simulink model "rockTrackingModelOne"  (R2023b)
settings: Solver=VariableStepAuto  StartTime=0.0  StopTime=10.0  RelTol=1e-3
settings Model: Creator=leif  LastModifiedBy=leif

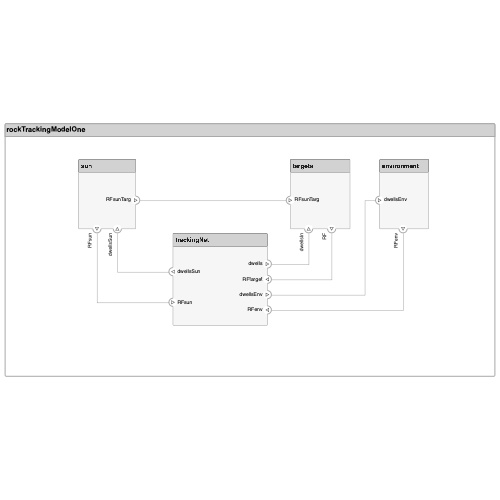
[thumbnail: Simulink's stored preview of the top-level diagram]
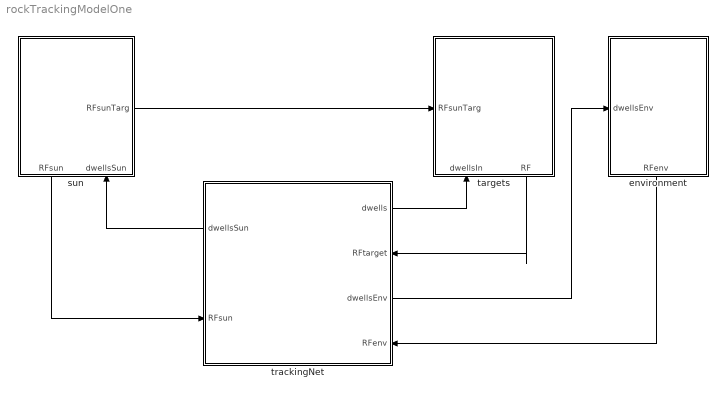
== system rockTrackingModelOne ==
  environment : Subsystem
      settings: PortSchema="{\"entries\":[{\"content\":{\"headerSize\":26,\"margin\":15,\"minimumSpacing\":25,\"sides\":[{\"content\":{\"connectorIds\":[\"In1\"]},\"type\":\"ConnectorPlacement.EquallySpacedRectSide\",\"uuid\":\"8862968b-5599-41d0-9291-c0c671b7ec34\"},{\"content\":{\"side\":\"RIGHT\"},\"type\":\"ConnectorPlacement.EquallySpacedRectSide\",\"uuid\":\"824bb606-5208-4b2e-9988-455833bc9c0f\"},{\"content\":{\"side\":\"TOP\"},\"type\":\"ConnectorPlacement.EquallySpacedRectSide\",\"uuid\":\"80947048-364c-4417-9b61-7a75165eca9d\"},{\"content\":{\"connectorIds\":[\"Out1\"],\"side\":\"BOTTOM\"},\"type\":\"ConnectorPlacement.EquallySpacedRectSide\",\"uuid\":\"629623b4-050a-43a5-9a7b-197cf824730b\"}]},\"type\":\"ConnectorPlacement.EquallySpacedConnector\",\"uuid\":\"bd0727a2-e7c6-4cf8-803d-4ba2eab1ab1b\"}],\"packageUris\":[\"http://schema.mathworks.com/mf0/Connector/R2020b\"],\"version\":\"1.0\"}"
  sun : Subsystem
      settings: PortSchema="{\"entries\":[{\"content\":{\"headerSize\":26,\"margin\":15,\"minimumSpacing\":25,\"sides\":[{\"content\":{},\"type\":\"ConnectorPlacement.EquallySpacedRectSide\",\"uuid\":\"8862968b-5599-41d0-9291-c0c671b7ec34\"},{\"content\":{\"connectorIds\":[\"Out2\"],\"side\":\"RIGHT\"},\"type\":\"ConnectorPlacement.EquallySpacedRectSide\",\"uuid\":\"824bb606-5208-4b2e-9988-455833bc9c0f\"},{\"content\":{\"side\":\"TOP\"},\"type\":\"ConnectorPlacement.EquallySpacedRectSide\",\"uuid\":\"80947048-364c-4417-9b61-7a75165eca9d\"},{\"content\":{\"connectorIds\":[\"Out1\",\"In1\"],\"side\":\"BOTTOM\"},\"type\":\"ConnectorPlacement.EquallySpacedRectSide\",\"uuid\":\"9527848b-f77a-4aa4-b4b8-8e4a885b14ab\"}]},\"type\":\"ConnectorPlacement.EquallySpacedConnector\",\"uuid\":\"bd0727a2-e7c6-4cf8-803d-4ba2eab1ab1b\"}],\"packageUris\":[\"http://schema.mathworks.com/mf0/Connector/R2020b\"],\"version\":\"1.0\"}"
  targets : Subsystem
      settings: PortSchema="{\"entries\":[{\"content\":{\"headerSize\":26,\"margin\":15,\"minimumSpacing\":25,\"sides\":[{\"content\":{\"connectorIds\":[\"In2\"]},\"type\":\"ConnectorPlacement.EquallySpacedRectSide\",\"uuid\":\"8862968b-5599-41d0-9291-c0c671b7ec34\"},{\"content\":{\"side\":\"RIGHT\"},\"type\":\"ConnectorPlacement.EquallySpacedRectSide\",\"uuid\":\"824bb606-5208-4b2e-9988-455833bc9c0f\"},{\"content\":{\"side\":\"TOP\"},\"type\":\"ConnectorPlacement.EquallySpacedRectSide\",\"uuid\":\"80947048-364c-4417-9b61-7a75165eca9d\"},{\"content\":{\"connectorIds\":[\"In1\",\"Out1\"],\"side\":\"BOTTOM\"},\"type\":\"ConnectorPlacement.EquallySpacedRectSide\",\"uuid\":\"629623b4-050a-43a5-9a7b-197cf824730b\"}]},\"type\":\"ConnectorPlacement.EquallySpacedConnector\",\"uuid\":\"bd0727a2-e7c6-4cf8-803d-4ba2eab1ab1b\"}],\"packageUris\":[\"http://schema.mathworks.com/mf0/Connector/R2020b\"],\"version\":\"1.0\"}"
  trackingNet : Subsystem
      settings: PortSchema="{\"entries\":[{\"content\":{\"headerSize\":26,\"margin\":15,\"minimumSpacing\":25,\"sides\":[{\"content\":{\"connectorIds\":[\"Out2\",\"In1\"]},\"type\":\"ConnectorPlacement.EquallySpacedRectSide\",\"uuid\":\"8862968b-5599-41d0-9291-c0c671b7ec34\"},{\"content\":{\"connectorIds\":[\"Out1\",\"In3\",\"Out3\",\"In2\"],\"side\":\"RIGHT\"},\"type\":\"ConnectorPlacement.EquallySpacedRectSide\",\"uuid\":\"824bb606-5208-4b2e-9988-455833bc9c0f\"},{\"content\":{\"side\":\"TOP\"},\"type\":\"ConnectorPlacement.EquallySpacedRectSide\",\"uuid\":\"80947048-364c-4417-9b61-7a75165eca9d\"}]},\"type\":\"ConnectorPlacement.EquallySpacedConnector\",\"uuid\":\"bd0727a2-e7c6-4cf8-803d-4ba2eab1ab1b\"}],\"packageUris\":[\"http://schema.mathworks.com/mf0/Connector/R2020b\"],\"version\":\"1.0\"}"
  wires:
  sun/2(RFsunTarg) -> targets/2(RFsunTarg)
  targets/1(RF) -> trackingNet/3(RFtarget)
  sun/1(RFsun) -> trackingNet/1(RFsun)
  trackingNet/3(dwellsEnv) -> environment/1(dwellsEnv)
  environment/1(RFenv) -> trackingNet/2(RFenv)
  trackingNet/2(dwellsSun) -> sun/1(dwellsSun)
  trackingNet/1(dwells) -> targets/1(dwellsIn)

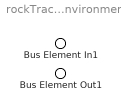
== system rockTrackingModelOne/environment ==
  Bus Element In1 : Inport  PortName=dwellsEnv
  Bus Element Out1 : Outport  PortName=RFenv

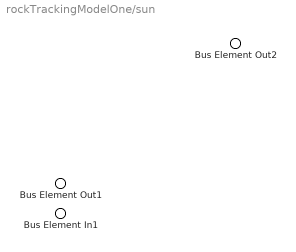
== system rockTrackingModelOne/sun ==
  Bus Element In1 : Inport  PortName=dwellsSun
  Bus Element Out2 : Outport  PortName=RFsun
  Bus Element Out1 : Outport  Port=2  PortName=RFsunTarg

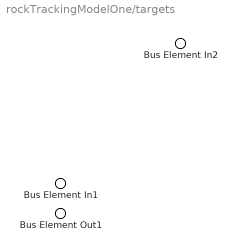
== system rockTrackingModelOne/targets ==
  Bus Element In2 : Inport  PortName=dwellsIn
  Bus Element In1 : Inport  Port=2  PortName=RFsunTarg
  Bus Element Out1 : Outport  PortName=RF

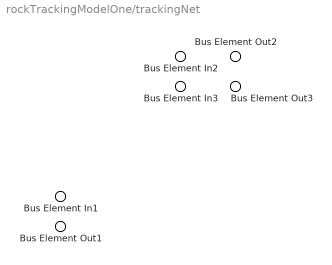
== system rockTrackingModelOne/trackingNet ==
  Bus Element In2 : Inport  PortName=RFsun
  Bus Element In3 : Inport  Port=2  PortName=RFenv
  Bus Element In1 : Inport  Port=3  PortName=RFtarget
  Bus Element Out3 : Outport  PortName=dwells
  Bus Element Out2 : Outport  Port=2  PortName=dwellsSun
  Bus Element Out1 : Outport  Port=3  PortName=dwellsEnv
